simulink model "GMCLIB_DecouplingPMSM_BAM_FLT"  (Simulink 7.3)
settings: Solver=ode45  StartTime=0.0  StopTime=10.0  RelTol=1e-3
undefined symbols (not defined in the file): fltKd, fltKq
settings Model: Creator=B17364  LastModifiedBy=B17364

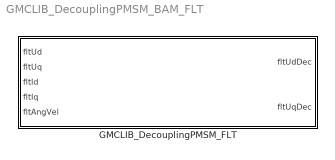
== system GMCLIB_DecouplingPMSM_BAM_FLT ==
  GMCLIB_DecouplingPMSM_FLT : Subsystem  mask(GMCLIB_DecouplingPMSM_FLT){fltKd=fltKd, fltKq=fltKq}
      mask help: Bit accurate model of decoupling for PMSM model.
      mask init:
      | pos = get_param(gcb, 'Position');width = pos(3) - pos(1); height = pos(4) - pos(2);tX=width/2;tY=height*0.9;
      mask Display: color('black');port_label('input',1,'fltUd');port_label('input',2,'fltUq');port_label('input',3,'fltId');port_label('input',4,'fltIq');port_label('input',5,'fltAngVel');port_label('output',1,'fltUdDec');port_label('output',2,'fltUqDec');color('black');disp('GMCLIB_DecouplingPMSM_FLT');color('blue');text(tX,tY, 'BAM', 'horizontalAlignment', 'center');

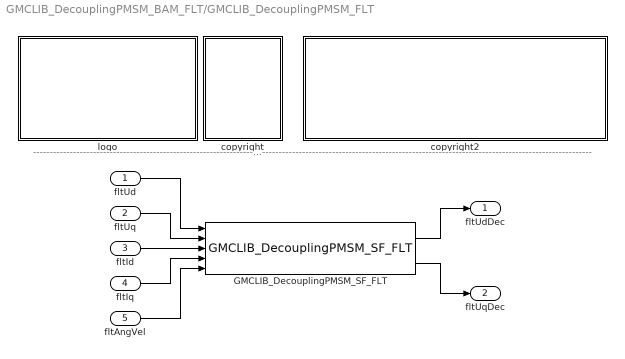
== system GMCLIB_DecouplingPMSM_BAM_FLT/GMCLIB_DecouplingPMSM_FLT ==
  note: ---------------------------------------------------------------------------------------------------------------------------------------------------------------------------------------------------
  fltUd : Inport  OutDataType=fixdt(1, 16)  OutScaling=2^0
  fltUq : Inport  Port=2  OutDataType=fixdt(1, 16)  OutScaling=2^0
  fltId : Inport  Port=3  OutDataType=fixdt(1, 16)  OutScaling=2^0
  fltIq : Inport  Port=4  OutDataType=fixdt(1, 16)  OutScaling=2^0
  fltAngVel : Inport  Port=5  OutDataType=fixdt(1, 16)  OutScaling=2^0
  GMCLIB_DecouplingPMSM_SF_FLT : S-Function  FunctionName=GMCLIB_DecouplingPMSM_SF_FLT  Parameters=fltKd,fltKq  EnableBusSupport=off
  copyright : Subsystem
      mask Display: text(10,90,'FILE:');text(10,75,'DESRIPTION:')text(10,60,'COPYRIGHT:')text(10,45,'VERSION:')text(10,30,'DATE:')
  copyright2 : Subsystem
      mask Display: text(10,90,'GMCLIB_DecouplingPMSM_BAM_FLT.mdl');text(10,75,'Decoupling of d and q axis of PMSM model.');text(10,60,'Freescale')text(10,45,'0.1');text(10,30,'14-Sep-2011');
  logo : Subsystem
      mask Display: image(imread('logo.jpg'))
  fltUdDec : Outport  OutDataType=fixdt(1, 16)  OutScaling=2^0
  fltUqDec : Outport  Port=2  OutDataType=fixdt(1, 16)  OutScaling=2^0
  wires:
  fltUd/1 -> GMCLIB_DecouplingPMSM_SF_FLT/1
  fltUq/1 -> GMCLIB_DecouplingPMSM_SF_FLT/2
  fltId/1 -> GMCLIB_DecouplingPMSM_SF_FLT/3
  fltIq/1 -> GMCLIB_DecouplingPMSM_SF_FLT/4
  fltAngVel/1 -> GMCLIB_DecouplingPMSM_SF_FLT/5
  GMCLIB_DecouplingPMSM_SF_FLT/1 -> fltUdDec/1
  GMCLIB_DecouplingPMSM_SF_FLT/2 -> fltUqDec/1

== system GMCLIB_DecouplingPMSM_BAM_FLT/GMCLIB_DecouplingPMSM_FLT/copyright ==

== system GMCLIB_DecouplingPMSM_BAM_FLT/GMCLIB_DecouplingPMSM_FLT/copyright2 ==

== system GMCLIB_DecouplingPMSM_BAM_FLT/GMCLIB_DecouplingPMSM_FLT/logo ==
